simulink model "RigidArmModel_3D"  (R2019a)
settings: Solver=VariableStepAuto  StartTime=0.0  StopTime=10  RelTol=1e-3
undefined symbols (not defined in the file): f_viscous, I1, I2, init_theta_1, init_theta_2, init_theta_dot_1, init_theta_dot_2, k1, k2, L1, L2, m1, m2, t1, t2, t_brk, t_c, theta_dot_brk, x_des, y_des
settings Model: Creator=Shaon  LastModifiedBy=Shaon

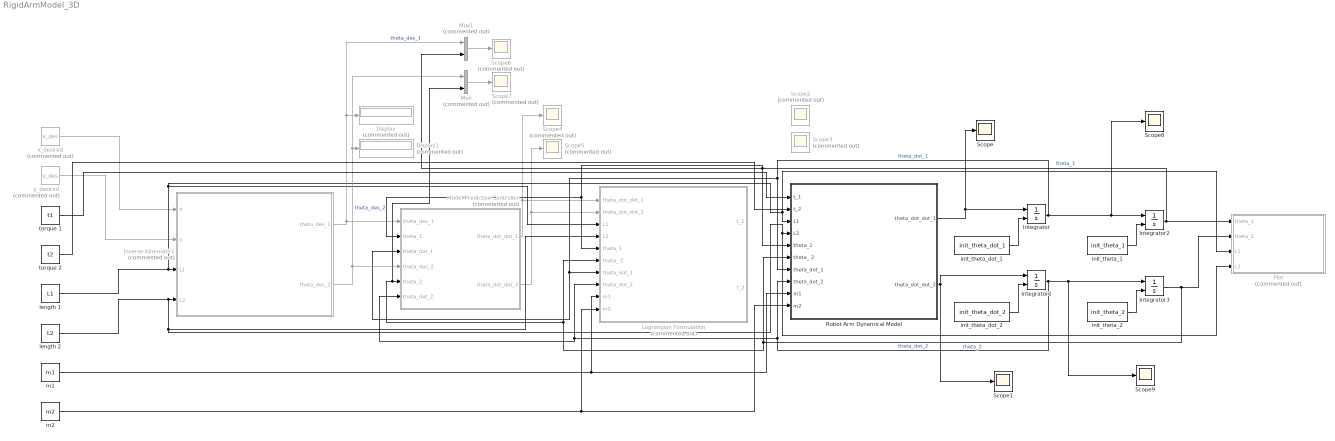
== system RigidArmModel_3D ==
  Display : Display  Commented=on
  Display1 : Display  Commented=on
  Integrator{,1..3} (4 alike) : Integrator  InitialConditionSource=external
  Inverse Kinematics : Subsystem  Commented=on
  Lagrangian Formulation : Subsystem  Commented=on
  Model Predictive Controller : Subsystem  Commented=on
  Mux : Mux  Commented=on  Inputs=2
  Mux1 : Mux  Commented=on  Inputs=2
  Plot : MATLAB Function  Commented=on  TreatAsAtomicUnit=on
  Robot Arm Dynamical Model : Subsystem
  Scope{,1,8..9} (4 alike) : Scope
  Scope{2..7} (6 alike) : Scope  Commented=on
  init_theta_1 : Constant  Value=init_theta_1
  init_theta_2 : Constant  Value=init_theta_2
  init_theta_dot_1 : Constant  Value=init_theta_dot_1
  init_theta_dot_2 : Constant  Value=init_theta_dot_2
  length 1 : Constant  Value=L1
  length 2 : Constant  Value=L2
  m1 : Constant  Value=m1
  m2 : Constant  Value=m2
  torque 1 : Constant  Value=t1
  torque 2 : Constant  Value=t2
  x_desired : Constant  Commented=on  Value=x_des
  y_desired : Constant  Commented=on  Value=y_des
  wires:
  Model Predictive Controller/1(theta_dot_dot_1) -> Scope4/1, Lagrangian Formulation/1(theta_dot_dot_1)
  Model Predictive Controller/2(theta_dot_dot_2) -> Scope5/1, Lagrangian Formulation/2(theta_dot_dot_2)
  init_theta_dot_1/1 -> Integrator/2
  Mux1/1 -> Scope6/1
  m2/1 -> Lagrangian Formulation/10(m2), Robot Arm Dynamical Model/10(m2)
  Robot Arm Dynamical Model/2(theta_dot_dot_2) -> Integrator1/1, Scope1/1
  m1/1 -> Lagrangian Formulation/9(m1), Robot Arm Dynamical Model/9(m1)
  x_desired/1 -> Inverse Kinematics/1(x)
  length 2/1 -> Lagrangian Formulation/4(L2), Plot/4(L2), Robot Arm Dynamical Model/4(L2), Inverse Kinematics/4(L2)
  y_desired/1 -> Inverse Kinematics/2(y)
  Integrator/1 -> Robot Arm Dynamical Model/7(theta_dot_1), Model Predictive Controller/3(theta_dot_1), Lagrangian Formulation/7(theta_dot_1), Scope8/1, Integrator2/1  "theta_dot_1"
  Mux/1 -> Scope7/1
  Integrator2/1 -> Robot Arm Dynamical Model/5("theta_1 "), Lagrangian Formulation/5("theta_1 "), Model Predictive Controller/2(theta_1), Mux1/2, Plot/1(theta_1)  "theta_1"
  Integrator1/1 -> Robot Arm Dynamical Model/8(theta_dot_2), Lagrangian Formulation/8(theta_dot_2), Model Predictive Controller/6(theta_dot_2), Scope9/1, Integrator3/1  "theta_dot_2"
  length 1/1 -> Lagrangian Formulation/3(L1), Plot/3(L1), Robot Arm Dynamical Model/3(L1), Inverse Kinematics/3(L1)
  Inverse Kinematics/1(theta_des_1) -> Model Predictive Controller/1(theta_des_1), Mux1/1, Display/1  "theta_des_1"
  Integrator3/1 -> Lagrangian Formulation/6(theta_ 2), Mux/2, Model Predictive Controller/5(theta_2), Robot Arm Dynamical Model/6(theta_ 2), Plot/2(theta_2)  "theta_2"
  Robot Arm Dynamical Model/1(theta_dot_dot_1) -> Scope/1, Integrator/1
  init_theta_1/1 -> Integrator2/2
  Inverse Kinematics/2(theta_des_2) -> Model Predictive Controller/4(theta_des_2), Mux/1, Display1/1  "theta_des_2"
  init_theta_dot_2/1 -> Integrator1/2
  init_theta_2/1 -> Integrator3/2
  torque 1/1 -> Robot Arm Dynamical Model/1(t_1)
  torque 2/1 -> Robot Arm Dynamical Model/2(t_2)

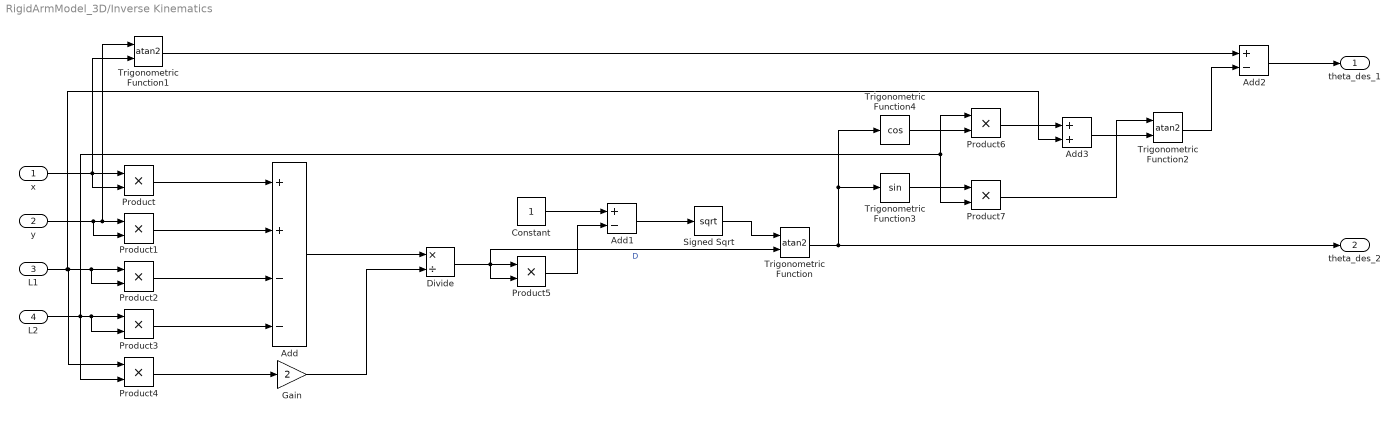
== system RigidArmModel_3D/Inverse Kinematics ==
  x : Inport
  y : Inport  Port=2
  L1 : Inport  Port=3
  L2 : Inport  Port=4
  Add : Sum  Inputs=++--
  Add1 : Sum  Inputs=+-
  Add2 : Sum  Inputs=+-
  Add3 : Sum
  Constant : Constant
  Divide : Product  Inputs=*/
  Gain : Gain  Gain=2
  Product{,1..7} (8 alike) : Product
  Signed Sqrt : Sqrt  SaturateOnIntegerOverflow=on
  Trigonometric Function : Trigonometry  Operator=atan2
  Trigonometric Function1 : Trigonometry  Operator=atan2
  Trigonometric Function2 : Trigonometry  Operator=atan2
  Trigonometric Function3 : Trigonometry
  Trigonometric Function4 : Trigonometry  Operator=cos
  theta_des_1 : Outport
  theta_des_2 : Outport  Port=2
  wires:
  Trigonometric Function2/1 -> Add2/2
  Trigonometric Function/1 -> theta_des_2/1, Trigonometric Function4/1, Trigonometric Function3/1
  Product1/1 -> Add/2
  Product/1 -> Add/1
  Trigonometric Function3/1 -> Product7/1
  y/1 -> Product1/1, Trigonometric Function1/1, Product1/2
  L2/1 -> Product6/1, Product7/2, Product4/2, Product3/2, Product3/1
  Trigonometric Function1/1 -> Add2/1
  Product6/1 -> Add3/1
  Trigonometric Function4/1 -> Product6/2
  Add2/1 -> theta_des_1/1
  Add3/1 -> Trigonometric Function2/2
  Constant/1 -> Add1/1
  L1/1 -> Add3/2, Product4/1, Product2/2, Product2/1
  Signed Sqrt/1 -> Trigonometric Function/1
  Add/1 -> Divide/1
  Product7/1 -> Trigonometric Function2/1
  x/1 -> Product/2, Product/1, Trigonometric Function1/2
  Product5/1 -> Add1/2
  Product2/1 -> Add/3
  Add1/1 -> Signed Sqrt/1
  Divide/1 -> Product5/2, Product5/1, Trigonometric Function/2  "D"
  Gain/1 -> Divide/2
  Product4/1 -> Gain/1
  Product3/1 -> Add/4

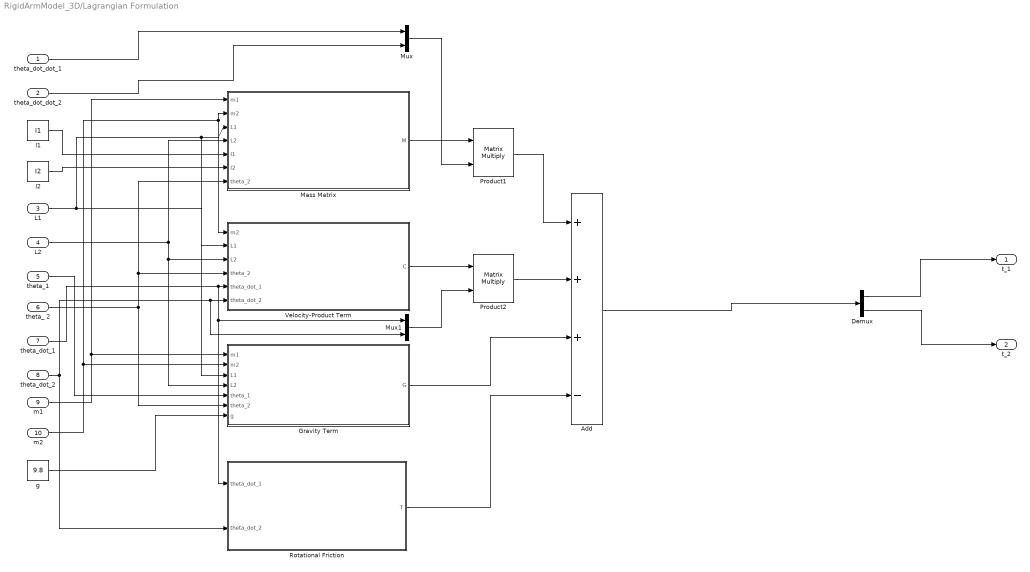
== system RigidArmModel_3D/Lagrangian Formulation ==
  theta_dot_dot_1 : Inport
  theta_dot_dot_2 : Inport  Port=2
  L1 : Inport  Port=3
  L2 : Inport  Port=4
  "theta_1 " : Inport  Port=5
  theta_ 2 : Inport  Port=6
  theta_dot_1 : Inport  Port=7
  theta_dot_2 : Inport  Port=8
  m1 : Inport  Port=9
  m2 : Inport  Port=10
  Add : Sum  Inputs=+++-
  Demux : Demux  Outputs=2
  Gravity Term : MATLAB Function  TreatAsAtomicUnit=on
  I1 : Constant  Value=I1
  I2 : Constant  Value=I2
  Mass Matrix : MATLAB Function  TreatAsAtomicUnit=on
  Mux : Mux  Inputs=2
  Mux1 : Mux  Inputs=2
  Product1 : Product  Multiplication=Matrix(*)
  Product2 : Product  Multiplication=Matrix(*)
  Rotational Friction : Subsystem
  Velocity-Product Term : MATLAB Function  TreatAsAtomicUnit=on
  g : Constant  Value=9.8
  t_1 : Outport
  t_2 : Outport  Port=2
  wires:
  Velocity-Product Term/1(C) -> Product2/1
  Gravity Term/1(G) -> Add/3
  Add/1 -> Demux/1
  Demux/1 -> t_1/1
  Demux/2 -> t_2/1
  theta_dot_dot_1/1 -> Mux/1
  theta_dot_dot_2/1 -> Mux/2
  m1/1 -> Gravity Term/1(m1), Mass Matrix/1(m1)
  m2/1 -> Gravity Term/2(m2), Velocity-Product Term/1(m2), Mass Matrix/2(m2)
  L1/1 -> Gravity Term/3(L1), Mass Matrix/3(L1), Velocity-Product Term/2(L1)
  L2/1 -> Velocity-Product Term/3(L2), Gravity Term/4(L2), Mass Matrix/4(L2)
  theta_ 2/1 -> Gravity Term/6(theta_2), Velocity-Product Term/4(theta_2), Mass Matrix/7(theta_2)
  theta_dot_1/1 -> Mux1/1, Rotational Friction/1("theta_dot_1 "), Velocity-Product Term/5(theta_dot_1)
  theta_dot_2/1 -> Rotational Friction/2(theta_dot_2), Velocity-Product Term/6(theta_dot_2), Mux1/2
  "theta_1 "/1 -> Gravity Term/5(theta_1)
  g/1 -> Gravity Term/7(g)
  Mass Matrix/1(M) -> Product1/1
  Mux/1 -> Product1/2
  Product1/1 -> Add/1
  I1/1 -> Mass Matrix/5(I1)
  I2/1 -> Mass Matrix/6(I2)
  Mux1/1 -> Product2/2
  Product2/1 -> Add/2
  Rotational Friction/1(T) -> Add/4

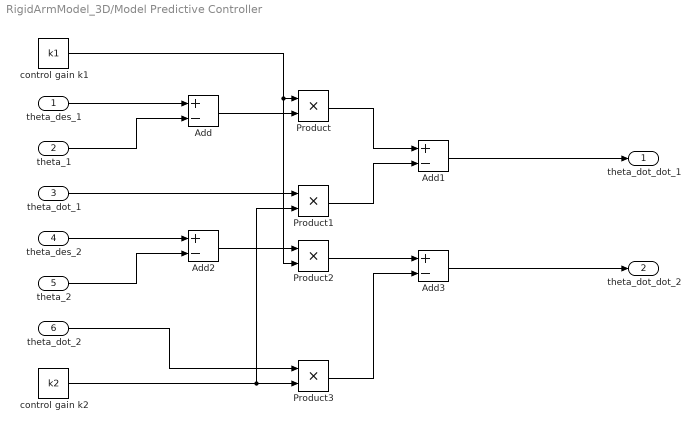
== system RigidArmModel_3D/Model Predictive Controller ==
  theta_des_1 : Inport
  theta_1 : Inport  Port=2
  theta_dot_1 : Inport  Port=3
  theta_des_2 : Inport  Port=4
  theta_2 : Inport  Port=5
  theta_dot_2 : Inport  Port=6
  Add{,1..3} (4 alike) : Sum  Inputs=+-
  Product{,1..3} (4 alike) : Product
  control gain k1 : Constant  Value=k1
  control gain k2 : Constant  Value=k2
  theta_dot_dot_1 : Outport
  theta_dot_dot_2 : Outport  Port=2
  wires:
  control gain k1/1 -> Product2/2, Product/1
  Product1/1 -> Add1/2
  Product3/1 -> Add3/2
  Add1/1 -> theta_dot_dot_1/1
  Add2/1 -> Product2/1
  Product/1 -> Add1/1
  theta_dot_2/1 -> Product3/1
  Add3/1 -> theta_dot_dot_2/1
  control gain k2/1 -> Product3/2, Product1/2
  Product2/1 -> Add3/1
  theta_2/1 -> Add2/2
  theta_dot_1/1 -> Product1/1
  theta_des_1/1 -> Add/1
  Add/1 -> Product/2
  theta_1/1 -> Add/2
  theta_des_2/1 -> Add2/1

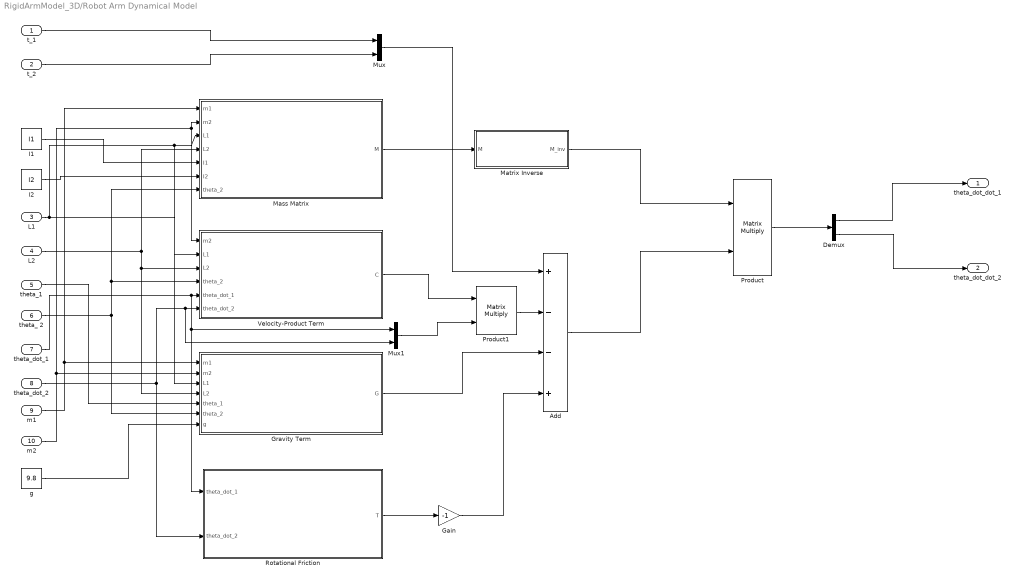
== system RigidArmModel_3D/Robot Arm Dynamical Model ==
  t_1 : Inport
  t_2 : Inport  Port=2
  L1 : Inport  Port=3
  L2 : Inport  Port=4
  "theta_1 " : Inport  Port=5
  theta_ 2 : Inport  Port=6
  theta_dot_1 : Inport  Port=7
  theta_dot_2 : Inport  Port=8
  m1 : Inport  Port=9
  m2 : Inport  Port=10
  Add : Sum  Inputs=+--+
  Demux : Demux  Outputs=2
  Gain : Gain  Gain=-1
  Gravity Term : MATLAB Function  TreatAsAtomicUnit=on
  I1 : Constant  Value=I1
  I2 : Constant  Value=I2
  Mass Matrix : MATLAB Function  TreatAsAtomicUnit=on
  Matrix Inverse : MATLAB Function  TreatAsAtomicUnit=on
  Mux : Mux  Inputs=2
  Mux1 : Mux  Inputs=2
  Product : Product  Multiplication=Matrix(*)
  Product1 : Product  Multiplication=Matrix(*)
  Rotational Friction : Subsystem
  Velocity-Product Term : MATLAB Function  TreatAsAtomicUnit=on
  g : Constant  Value=9.8
  theta_dot_dot_1 : Outport
  theta_dot_dot_2 : Outport  Port=2
  wires:
  Mux/1 -> Add/1
  Velocity-Product Term/1(C) -> Product1/1
  Gravity Term/1(G) -> Add/3
  Mass Matrix/1(M) -> Matrix Inverse/1(M)
  Matrix Inverse/1(M_inv) -> Product/1
  Add/1 -> Product/2
  Product/1 -> Demux/1
  Demux/1 -> theta_dot_dot_1/1
  Demux/2 -> theta_dot_dot_2/1
  t_1/1 -> Mux/1
  t_2/1 -> Mux/2
  m1/1 -> Gravity Term/1(m1), Mass Matrix/1(m1)
  m2/1 -> Gravity Term/2(m2), Velocity-Product Term/1(m2), Mass Matrix/2(m2)
  L1/1 -> Gravity Term/3(L1), Mass Matrix/3(L1), Velocity-Product Term/2(L1)
  L2/1 -> Velocity-Product Term/3(L2), Gravity Term/4(L2), Mass Matrix/4(L2)
  theta_ 2/1 -> Gravity Term/6(theta_2), Velocity-Product Term/4(theta_2), Mass Matrix/7(theta_2)
  theta_dot_1/1 -> Mux1/1, Rotational Friction/1("theta_dot_1 "), Velocity-Product Term/5(theta_dot_1)
  theta_dot_2/1 -> Rotational Friction/2(theta_dot_2), Velocity-Product Term/6(theta_dot_2), Mux1/2
  "theta_1 "/1 -> Gravity Term/5(theta_1)
  g/1 -> Gravity Term/7(g)
  I1/1 -> Mass Matrix/5(I1)
  I2/1 -> Mass Matrix/6(I2)
  Product1/1 -> Add/2
  Mux1/1 -> Product1/2
  Gain/1 -> Add/4
  Rotational Friction/1(T) -> Gain/1

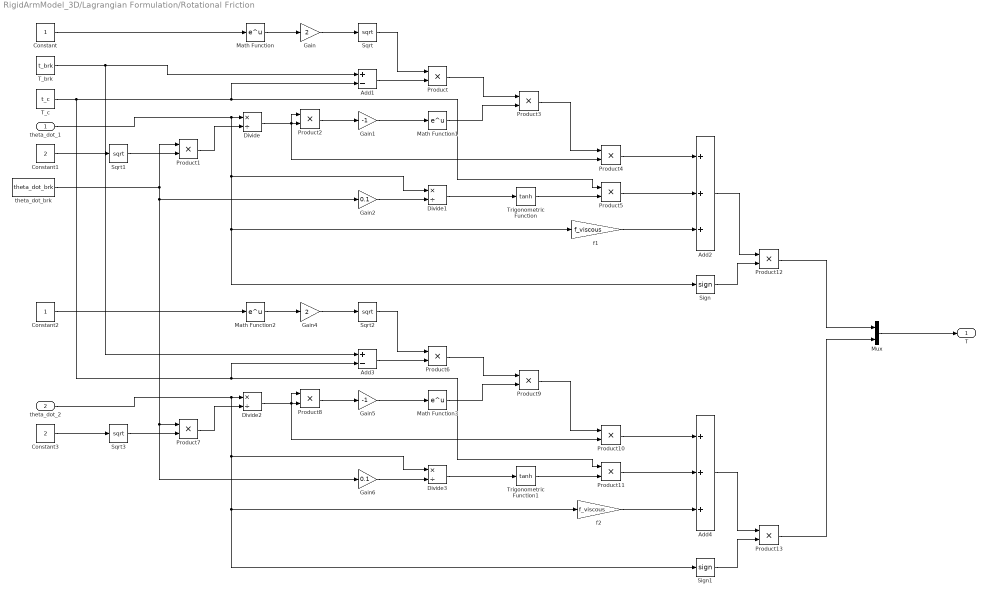
== system RigidArmModel_3D/Lagrangian Formulation/Rotational Friction ==
  "theta_dot_1 " : Inport
  theta_dot_2 : Inport  Port=2
  Add1 : Sum  Inputs=+-
  Add2 : Sum  Inputs=+++
  Add3 : Sum  Inputs=+-
  Add4 : Sum  Inputs=+++
  Constant : Constant
  Constant1 : Constant  Value=2
  Constant2 : Constant
  Constant3 : Constant  Value=2
  Divide{,1..3} (4 alike) : Product  Inputs=*/
  Gain : Gain  Gain=2
  Gain1 : Gain  Gain=-1
  Gain2 : Gain  Gain=0.1
  Gain4 : Gain  Gain=2
  Gain5 : Gain  Gain=-1
  Gain6 : Gain  Gain=0.1
  Math Function{,1..3} (4 alike) : Math  SaturateOnIntegerOverflow=on
  Mux : Mux  Inputs=2
  Product{,1..13} (14 alike) : Product
  Sign : Signum
  Sign1 : Signum
  Sqrt{,1..3} (4 alike) : Sqrt  SaturateOnIntegerOverflow=on
  T_brk : Constant  Value=t_brk
  T_c : Constant  Value=t_c
  Trigonometric Function : Trigonometry  Operator=tanh
  Trigonometric Function1 : Trigonometry  Operator=tanh
  f1 : Gain  Gain=f_viscous
  f2 : Gain  Gain=f_viscous
  theta_dot_brk : Constant  Value=theta_dot_brk
  T : Outport
  wires:
  Math Function/1 -> Gain/1
  Sqrt/1 -> Product/1
  Gain/1 -> Sqrt/1
  Constant/1 -> Math Function/1
  Product3/1 -> Product4/1
  Product/1 -> Product3/1
  Add1/1 -> Product/2
  Math Function1/1 -> Product3/2
  "theta_dot_1 "/1 -> Sign/1, f1/1, Divide1/1, Divide/1
  Constant1/1 -> Sqrt1/1
  Sqrt1/1 -> Product1/2
  Product1/1 -> Divide/2
  Divide/1 -> Product2/1, Product2/2, Product4/2
  Product2/1 -> Gain1/1
  Gain1/1 -> Math Function1/1
  Product4/1 -> Add2/1
  Divide1/1 -> Trigonometric Function/1
  Gain2/1 -> Divide1/2
  Trigonometric Function/1 -> Product5/2
  Product5/1 -> Add2/2
  f1/1 -> Add2/3
  Add2/1 -> Product12/1
  T_brk/1 -> Add3/1, Add1/1
  Add3/1 -> Product6/2
  Product9/1 -> Product10/1
  Divide2/1 -> Product8/1, Product8/2, Product10/2
  Product7/1 -> Divide2/2
  Constant3/1 -> Sqrt3/1
  Product8/1 -> Gain5/1
  theta_dot_brk/1 -> Gain6/1, Product7/1, Gain2/1, Product1/1
  Divide3/1 -> Trigonometric Function1/1
  Gain5/1 -> Math Function3/1
  theta_dot_2/1 -> Divide3/1, Sign1/1, f2/1, Divide2/1
  Product10/1 -> Add4/1
  Product6/1 -> Product9/1
  Gain6/1 -> Divide3/2
  Product13/1 -> Mux/2
  Trigonometric Function1/1 -> Product11/2
  Math Function3/1 -> Product9/2
  Gain4/1 -> Sqrt2/1
  T_c/1 -> Product11/1, Add3/2, Product5/1, Add1/2
  Math Function2/1 -> Gain4/1
  Constant2/1 -> Math Function2/1
  Sqrt2/1 -> Product6/1
  Product11/1 -> Add4/2
  f2/1 -> Add4/3
  Sqrt3/1 -> Product7/2
  Mux/1 -> T/1
  Sign/1 -> Product12/2
  Product12/1 -> Mux/1
  Add4/1 -> Product13/1
  Sign1/1 -> Product13/2

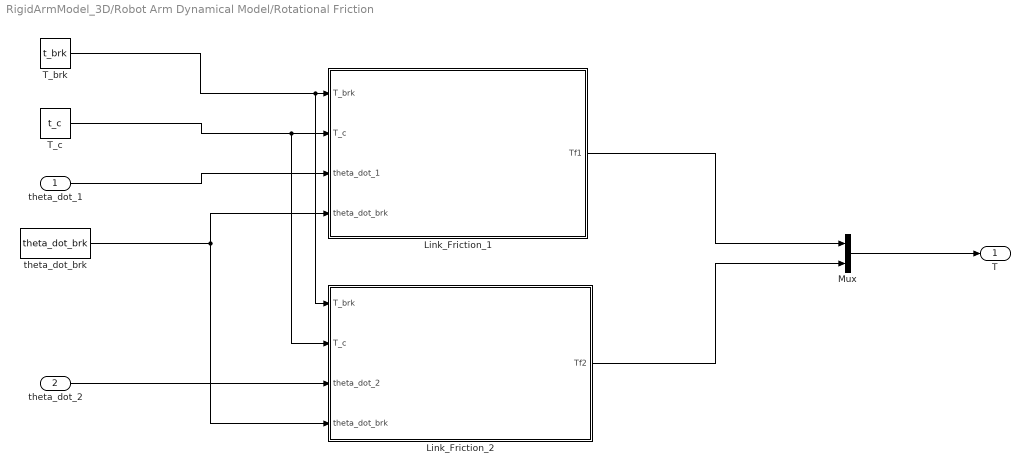
== system RigidArmModel_3D/Robot Arm Dynamical Model/Rotational Friction ==
  "theta_dot_1 " : Inport
  theta_dot_2 : Inport  Port=2
  Link_Friction_1 : Subsystem
  Link_Friction_2 : Subsystem
  Mux : Mux  Inputs=2
  T_brk : Constant  Value=t_brk
  T_c : Constant  Value=t_c
  theta_dot_brk : Constant  Value=theta_dot_brk
  T : Outport
  wires:
  Mux/1 -> T/1
  T_brk/1 -> Link_Friction_2/1(T_brk), Link_Friction_1/1(T_brk)
  T_c/1 -> Link_Friction_1/2(T_c), Link_Friction_2/2(T_c)
  "theta_dot_1 "/1 -> Link_Friction_1/3(theta_dot_1)
  theta_dot_brk/1 -> Link_Friction_2/4(theta_dot_brk), Link_Friction_1/4(theta_dot_brk)
  Link_Friction_1/1(Tf1) -> Mux/1
  theta_dot_2/1 -> Link_Friction_2/3(theta_dot_2)
  Link_Friction_2/1(Tf2) -> Mux/2

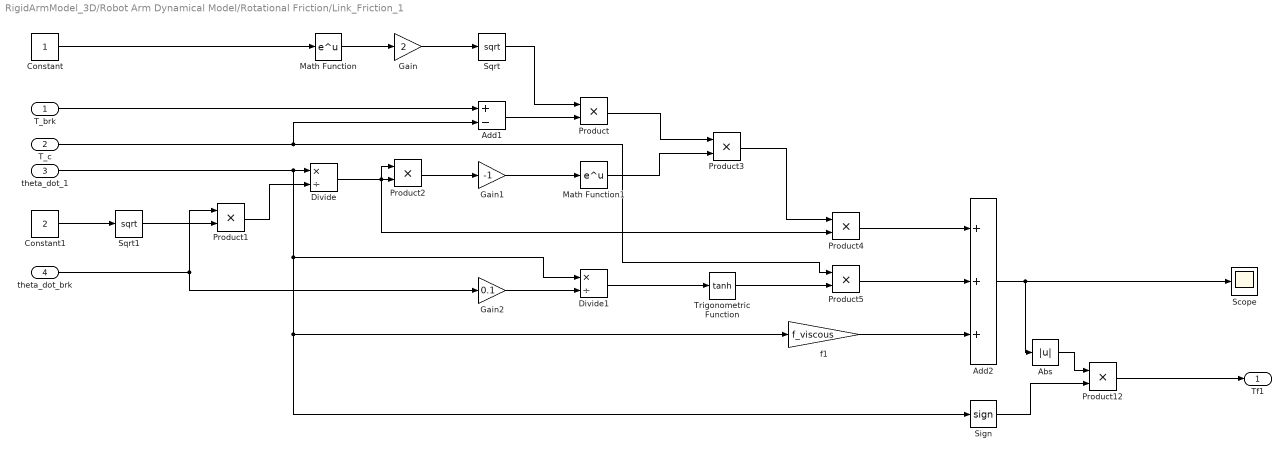
== system RigidArmModel_3D/Robot Arm Dynamical Model/Rotational Friction/Link_Friction_1 ==
  T_brk : Inport
  T_c : Inport  Port=2
  theta_dot_1 : Inport  Port=3
  theta_dot_brk : Inport  Port=4
  Abs : Abs
  Add1 : Sum  Inputs=+-
  Add2 : Sum  Inputs=+++
  Constant : Constant
  Constant1 : Constant  Value=2
  Divide : Product  Inputs=*/
  Divide1 : Product  Inputs=*/
  Gain : Gain  Gain=2
  Gain1 : Gain  Gain=-1
  Gain2 : Gain  Gain=0.1
  Math Function : Math  SaturateOnIntegerOverflow=on
  Math Function1 : Math  SaturateOnIntegerOverflow=on
  Product{,1..5,12} (7 alike) : Product
  Scope : Scope
  Sign : Signum
  Sqrt : Sqrt  SaturateOnIntegerOverflow=on
  Sqrt1 : Sqrt  SaturateOnIntegerOverflow=on
  Trigonometric Function : Trigonometry  Operator=tanh
  f1 : Gain  Gain=f_viscous
  Tf1 : Outport
  wires:
  Gain/1 -> Sqrt/1
  Product5/1 -> Add2/2
  Divide1/1 -> Trigonometric Function/1
  Constant1/1 -> Sqrt1/1
  theta_dot_1/1 -> Sign/1, f1/1, Divide1/1, Divide/1
  Add1/1 -> Product/2
  Divide/1 -> Product2/1, Product2/2, Product4/2
  Constant/1 -> Math Function/1
  Add2/1 -> Abs/1, Scope/1
  Product3/1 -> Product4/1
  Gain1/1 -> Math Function1/1
  Trigonometric Function/1 -> Product5/2
  Abs/1 -> Product12/1
  f1/1 -> Add2/3
  Math Function/1 -> Gain/1
  Product4/1 -> Add2/1
  Gain2/1 -> Divide1/2
  Sqrt/1 -> Product/1
  Sign/1 -> Product12/2
  Product/1 -> Product3/1
  Product2/1 -> Gain1/1
  Product1/1 -> Divide/2
  T_c/1 -> Product5/1, Add1/2
  Math Function1/1 -> Product3/2
  theta_dot_brk/1 -> Gain2/1, Product1/1
  T_brk/1 -> Add1/1
  Sqrt1/1 -> Product1/2
  Product12/1 -> Tf1/1

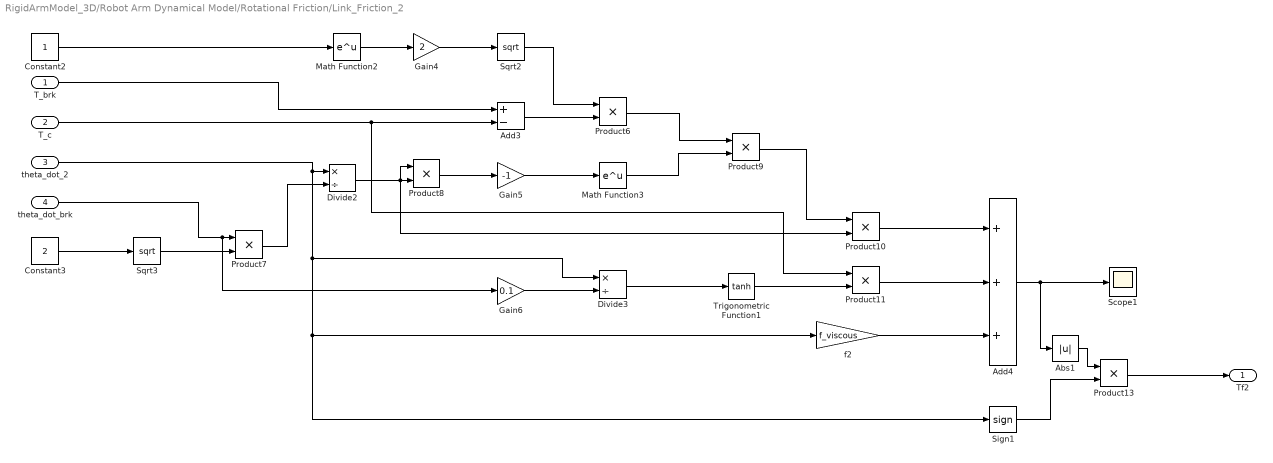
== system RigidArmModel_3D/Robot Arm Dynamical Model/Rotational Friction/Link_Friction_2 ==
  T_brk : Inport
  T_c : Inport  Port=2
  theta_dot_2 : Inport  Port=3
  theta_dot_brk : Inport  Port=4
  Abs1 : Abs
  Add3 : Sum  Inputs=+-
  Add4 : Sum  Inputs=+++
  Constant2 : Constant
  Constant3 : Constant  Value=2
  Divide2 : Product  Inputs=*/
  Divide3 : Product  Inputs=*/
  Gain4 : Gain  Gain=2
  Gain5 : Gain  Gain=-1
  Gain6 : Gain  Gain=0.1
  Math Function2 : Math  SaturateOnIntegerOverflow=on
  Math Function3 : Math  SaturateOnIntegerOverflow=on
  Product{6..11,13} (7 alike) : Product
  Scope1 : Scope
  Sign1 : Signum
  Sqrt2 : Sqrt  SaturateOnIntegerOverflow=on
  Sqrt3 : Sqrt  SaturateOnIntegerOverflow=on
  Trigonometric Function1 : Trigonometry  Operator=tanh
  f2 : Gain  Gain=f_viscous
  Tf2 : Outport
  wires:
  Add3/1 -> Product6/2
  Product9/1 -> Product10/1
  Product10/1 -> Add4/1
  Sign1/1 -> Product13/2
  Product7/1 -> Divide2/2
  Divide2/1 -> Product8/1, Product8/2, Product10/2
  theta_dot_2/1 -> Divide3/1, Sign1/1, f2/1, Divide2/1
  Math Function3/1 -> Product9/2
  Gain5/1 -> Math Function3/1
  Constant3/1 -> Sqrt3/1
  Math Function2/1 -> Gain4/1
  Add4/1 -> Abs1/1, Scope1/1
  theta_dot_brk/1 -> Gain6/1, Product7/1
  Gain6/1 -> Divide3/2
  Product6/1 -> Product9/1
  Product8/1 -> Gain5/1
  Sqrt3/1 -> Product7/2
  Abs1/1 -> Product13/1
  Constant2/1 -> Math Function2/1
  Sqrt2/1 -> Product6/1
  f2/1 -> Add4/3
  Gain4/1 -> Sqrt2/1
  Product11/1 -> Add4/2
  Divide3/1 -> Trigonometric Function1/1
  Trigonometric Function1/1 -> Product11/2
  T_brk/1 -> Add3/1
  T_c/1 -> Product11/1, Add3/2
  Product13/1 -> Tf2/1

== matlab function RigidArmModel_3D/Robot Arm Dynamical Model/Velocity-Product Term ==
  data: m2 input; C output size=[2,2]; L1 input; L2 input; theta_2 input; theta_dot_1 input; theta_dot_2 input
function C = velocity_product(m2, L1, L2, theta_2, theta_dot_1, theta_dot_2)
    %#codegen
    Lc2 = L2 / 2;
    h = -m2 * L1 * Lc2 * sin(theta_2);
    
    C_11 = h * theta_dot_2;
    C_12 = h * theta_dot_2 + h * theta_dot_1;
    C_21 = -h * theta_dot_1;
    C_22 = 0;
    
    C = [C_11 C_12; C_21 C_22];
end

== matlab function RigidArmModel_3D/Robot Arm Dynamical Model/Mass Matrix ==
  data: m1 input; M output size=[2,2]; m2 input; L1 input; L2 input; I1 input; I2 input; theta_2 input
function M = mass_matrix(m1, m2, L1, L2,I1, I2, theta_2)
    %#codegen
    Lc1 = L1 / 2;
    Lc2 = L2 / 2;
    
    M_11 = m1 * Lc1^2 + m2 * (L1^2 + Lc2^2 + 2 * L1 * Lc2 * cos(theta_2)) + I1 + I2;
    M_12 = m2 * (L1 * Lc2 * cos(theta_2) + Lc2^2) + I2;
    M_21 = m2 * (L1 * Lc2 * cos(theta_2) + Lc2^2) + I2;
    M_22 = m2 * Lc2^2 + I2;
    
    M = [M_11 M_12; M_21 M_22];
end

== matlab function RigidArmModel_3D/Robot Arm Dynamical Model/Gravity Term ==
  data: m1 input; G output size=[2,1]; m2 input; L1 input; L2 input; theta_1 input; theta_2 input; g input
function G = gravity(m1, m2, L1, L2, theta_1, theta_2, g)
    %#codegen
    Lc1 = L1 / 2;
    Lc2 = L2 / 2;
    
    G_11 = (m1 * Lc1 + m2 * L1) * g * cos(theta_1) + m2 * Lc2 * g * cos(theta_1 + theta_2);
    G_21 = m2 * g * Lc2 * cos(theta_1 + theta_2);
    
    G = [G_11; G_21];
end

== matlab function RigidArmModel_3D/Robot Arm Dynamical Model/Matrix Inverse ==
  data: M input size=[2,2]; M_inv output size=[2,2]
function M_inv = matrix_inv(M)
    M_inv = inv(M);
end

== matlab function RigidArmModel_3D/Plot ==
  data: theta_1 input; theta_2 input; L1 input; L2 input
function create_plot(theta_1, theta_2, L1, L2)
    coder.extrinsic('plot');

    x0 = 0;
    y0 = 0;
    x1 = L1 * cos(theta_1);
    y1 = L1 * sin(theta_1);
    x2 = L1 * cos(theta_1) + L2 * cos(theta_1 + theta_2);
    y2 = L1 * sin(theta_1) + L2 * sin(theta_1 + theta_2);
    
    clf;
    plot(0, 0, 's', 'MarkerFaceColor', 'red');
    hold on
    plot(x1, y1, 'o', 'MarkerFaceColor', 'green');
    hold on
    plot([x0 x1 x2], [y0 y1 y2]);
    
%     plot([x0 x1 x2], [y0 y1 y2], '-o', 'MarkerFaceColor', 'red');
    xlim([-2 2]);
    ylim([-2 2]);
    axis('equal');
end

== matlab function RigidArmModel_3D/Lagrangian Formulation/Gravity Term ==
  data: m1 input; G output size=[2,1]; m2 input; L1 input; L2 input; theta_1 input; theta_2 input; g input
function G = gravity(m1, m2, L1, L2, theta_1, theta_2, g)
    %#codegen
    Lc1 = L1 / 2;
    Lc2 = L2 / 2;
    
    G_11 = (m1 * Lc1 + m2 * L1) * g * cos(theta_1) + m2 * Lc2 * g * cos(theta_1 + theta_2);
    G_21 = m2 * g * Lc2 * cos(theta_1 + theta_2);
    
    G = [G_11; G_21];
end

== matlab function RigidArmModel_3D/Lagrangian Formulation/Mass Matrix ==
  data: m1 input; M output size=[2,2]; m2 input; L1 input; L2 input; I1 input; I2 input; theta_2 input
function M = mass_matrix(m1, m2, L1, L2,I1, I2, theta_2)
    %#codegen
    Lc1 = L1 / 2;
    Lc2 = L2 / 2;
    
    M_11 = m1 * Lc1^2 + m2 * (L1^2 + Lc2^2 + 2 * L1 * Lc2 * cos(theta_2)) + I1 + I2;
    M_12 = m2 * (L1 * Lc2 * cos(theta_2) + Lc2^2) + I2;
    M_21 = m2 * (L1 * Lc2 * cos(theta_2) + Lc2^2) + I2;
    M_22 = m2 * Lc2^2 + I2;
    
    M = [M_11 M_12; M_21 M_22];
end

== matlab function RigidArmModel_3D/Lagrangian Formulation/Velocity-Product Term ==
  data: m2 input; C output size=[2,2]; L1 input; L2 input; theta_2 input; theta_dot_1 input; theta_dot_2 input
function C = velocity_product(m2, L1, L2, theta_2, theta_dot_1, theta_dot_2)
    %#codegen
    Lc2 = L2 / 2;
    h = -m2 * L1 * Lc2 * sin(theta_2);
    
    C_11 = h * theta_dot_2;
    C_12 = h * theta_dot_2 + h * theta_dot_1;
    C_21 = -h * theta_dot_1;
    C_22 = 0;
    
    C = [C_11 C_12; C_21 C_22];
end
